simulink model "AtomicSubsystem"  (R2022b)
settings: Solver=VariableStepAuto  StartTime=0.0  StopTime=10.0  RelTol=1e-3
settings Model: Creator=Brigosha_Guest  LastModifiedBy=Brigosha_Guest

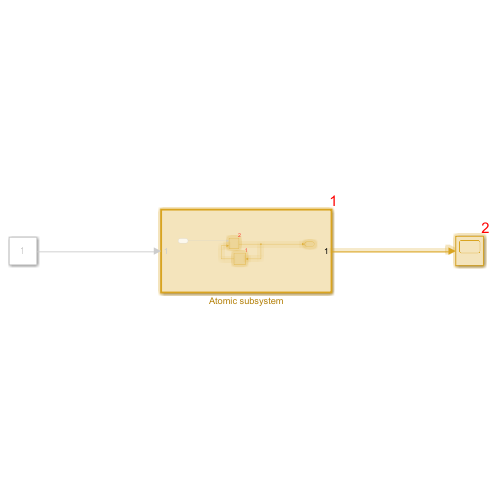
[thumbnail: Simulink's stored preview of the top-level diagram]
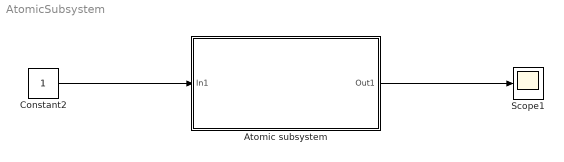
== system AtomicSubsystem ==
  Atomic subsystem : Subsystem  TreatAsAtomicUnit=on
  Constant2 : Constant
  Scope1 : Scope
  wires:
  Atomic subsystem/1(Out1) -> Scope1/1
  Constant2/1 -> Atomic subsystem/1(In1)

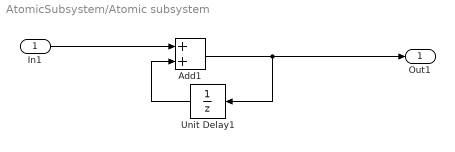
== system AtomicSubsystem/Atomic subsystem ==
  In1 : Inport
  Add1 : Sum
  Unit Delay1 : UnitDelay  SampleTime=-1  HasFrameUpgradeWarning=on
  Out1 : Outport
  wires:
  Unit Delay1/1 -> Add1/2
  In1/1 -> Add1/1
  Add1/1 -> Unit Delay1/1, Out1/1
